simulink model "ECE724A"  (R2021b)
settings: Solver=ode3  StartTime=0.0  StopTime=sim_duration  FixedStep=0.01  RelTol=1e-3
model workspace: external: MAT-File C:\Users\jimmy\Desktop\61508010.mat (data not in the file)
undefined symbols (not defined in the file or in its folder): Base_power, columbeff, efficiency, efficiency_speed, efficiency_torque, f_d, f_tire_friction, f_tire_speed, g, gear_efficiency, Init_capacity, J_fd, J_motor, J_wheel, OCV, OCV_SOC, R_chg, R_dis, r_mass, Regen_fraction, Regen_speed, Road_grade, SOC_init, SOC_min, Stop_speed, Torque_curve_speed, Torque_curve_torque, Vehicle_weight, Wheel_radius
libraries: simulink x1
settings Model: Creator=jimmy  LastModifiedBy=jimmy

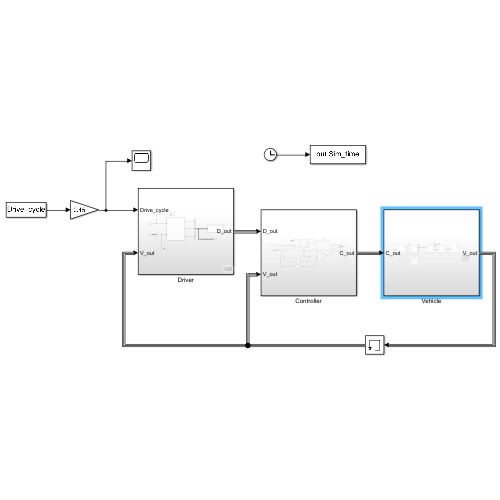
[thumbnail: Simulink's stored preview of the top-level diagram]
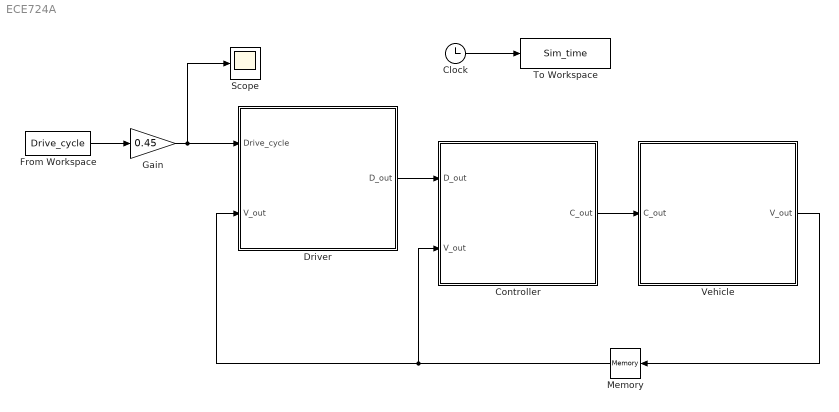
== system ECE724A ==
  Clock : Clock
  Controller : Subsystem
  Driver : Subsystem
  From Workspace : FromWorkspace  VariableName=Drive_cycle
  Gain : Gain  Gain=0.45
  Memory : Memory  InheritSampleTime=on  LinearizeMemory=on  LinearizeAsDelay=on
  Scope : Scope
  To Workspace : ToWorkspace  VariableName=Sim_time  SaveFormat=Timeseries  SampleTime=-1
  Vehicle : Subsystem
  wires:
  Vehicle/1(V_out) -> Memory/1
  Controller/1(C_out) -> Vehicle/1(C_out)
  Memory/1 -> Controller/2(V_out), Driver/2(V_out)
  Clock/1 -> To Workspace/1
  Driver/1(D_out) -> Controller/1(D_out)
  From Workspace/1 -> Gain/1
  Gain/1 -> Scope/1, Driver/1(Drive_cycle)

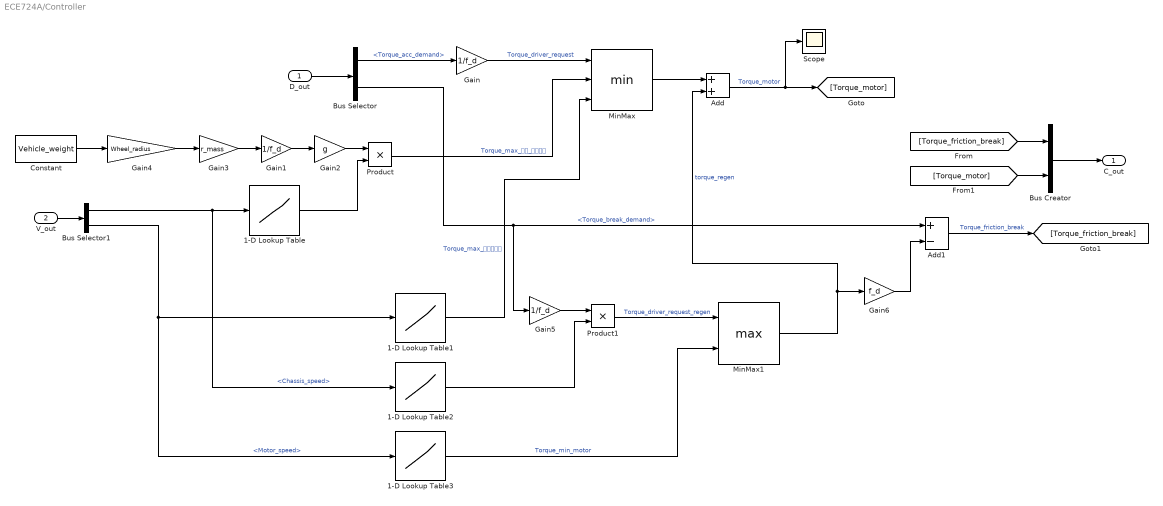
== system ECE724A/Controller ==
  D_out : Inport
  V_out : Inport  Port=2
  1-D Lookup Table : Lookup_n-D  NumberOfTableDimensions=1  BreakpointsForDimension1=f_tire_speed  Table=f_tire_friction  InternalRulePriority=Speed  RndMeth=Simplest  InputSameDT=on
  1-D Lookup Table1 : Lookup_n-D  NumberOfTableDimensions=1  BreakpointsForDimension1=Torque_curve_speed  Table=Torque_curve_torque  InternalRulePriority=Speed  RndMeth=Simplest  InputSameDT=on
  1-D Lookup Table2 : Lookup_n-D  NumberOfTableDimensions=1  BreakpointsForDimension1=Regen_speed  Table=Regen_fraction  InternalRulePriority=Speed  RndMeth=Simplest  InputSameDT=on
  1-D Lookup Table3 : Lookup_n-D  NumberOfTableDimensions=1  BreakpointsForDimension1=Torque_curve_speed  Table=-Torque_curve_torque  InternalRulePriority=Speed  RndMeth=Simplest  InputSameDT=on
  Add : Sum
  Add1 : Sum  Inputs=+-
  Bus Creator : BusCreator  Inputs=2
  Bus Selector : BusSelector  OutputSignals=Torque_acc_demand,Torque_break_demand
  Bus Selector1 : BusSelector  OutputSignals=Chassis.Chassis_speed,Motor.Motor_speed
  Constant : Constant  Value=Vehicle_weight
  Gain : Gain  Gain=1/f_d
  Gain1 : Gain  Gain=1/f_d
  Gain2 : Gain  Gain=g
  Gain3 : Gain  Gain=r_mass
  Gain4 : Gain  Gain=Wheel_radius
  Gain5 : Gain  Gain=1/f_d
  Gain6 : Gain  Gain=f_d
  MinMax : MinMax  Inputs=3
  MinMax1 : MinMax  Function=max  Inputs=2
  Product : Product
  Product1 : Product
  Scope : Scope
  C_out : Outport
  wires:
  D_out/1 -> Bus Selector/1
  Bus Selector/1 -> Gain/1  "<Torque_acc_demand>"
  Bus Selector/2 -> Gain5/1, Add1/1  "<Torque_break_demand>"
  Gain/1 -> MinMax/1  "Torque_driver_request"
  Constant/1 -> Gain4/1
  Gain4/1 -> Gain3/1
  Gain3/1 -> Gain1/1
  Gain1/1 -> Gain2/1
  1-D Lookup Table/1 -> Product/2
  Bus Selector1/1 -> 1-D Lookup Table2/1, 1-D Lookup Table/1  "<Chassis_speed>"
  Gain2/1 -> Product/1
  V_out/1 -> Bus Selector1/1
  Product/1 -> MinMax/2  "Torque_max_𝑛𝑜_𝑠𝑙𝑖𝑝"
  MinMax/1 -> Add/1
  Bus Selector1/2 -> 1-D Lookup Table3/1, 1-D Lookup Table1/1  "<Motor_speed>"
  1-D Lookup Table1/1 -> MinMax/3  "Torque_max_𝑚𝑜𝑡𝑜𝑟"
  Gain5/1 -> Product1/1
  1-D Lookup Table2/1 -> Product1/2
  Product1/1 -> MinMax1/1  "Torque_driver_request_regen"
  1-D Lookup Table3/1 -> MinMax1/2  "Torque_min_motor"
  MinMax1/1 -> Gain6/1, Add/2  "torque_regen"
  Add/1 -> Scope/1, [Torque_motor]  "Torque_motor"
  Gain6/1 -> Add1/2
  Add1/1 -> [Torque_friction_break]  "Torque_friction_break"
  [Torque_motor] -> Bus Creator/2
  [Torque_friction_break] -> Bus Creator/1
  Bus Creator/1 -> C_out/1

== system ECE724A/Driver ==
  Drive_cycle : Inport
  V_out : Inport  Port=2
  Bus Creator : BusCreator  Inputs=3
  Bus Selector : BusSelector  OutputSignals=Chassis.Chassis_speed
  Plant : Subsystem
  Scope : Scope
  Scope1 : Scope
  To workspace : Subsystem
  D_out : Outport
  wires:
  Drive_cycle/1 -> Scope/1, Plant/1(Drive_cycle)
  V_out/1 -> Bus Selector/1
  Bus Selector/1 -> Scope1/1, Plant/2(Chasis_speed)  "<Chassis_speed>"
  Plant/1(Linear_speed_demand) -> Bus Creator/1
  Plant/2(Torque_acc_demand) -> Bus Creator/2
  Plant/3(Torque_break_demand) -> Bus Creator/3
  Bus Creator/1 -> D_out/1, To workspace/1(In1)

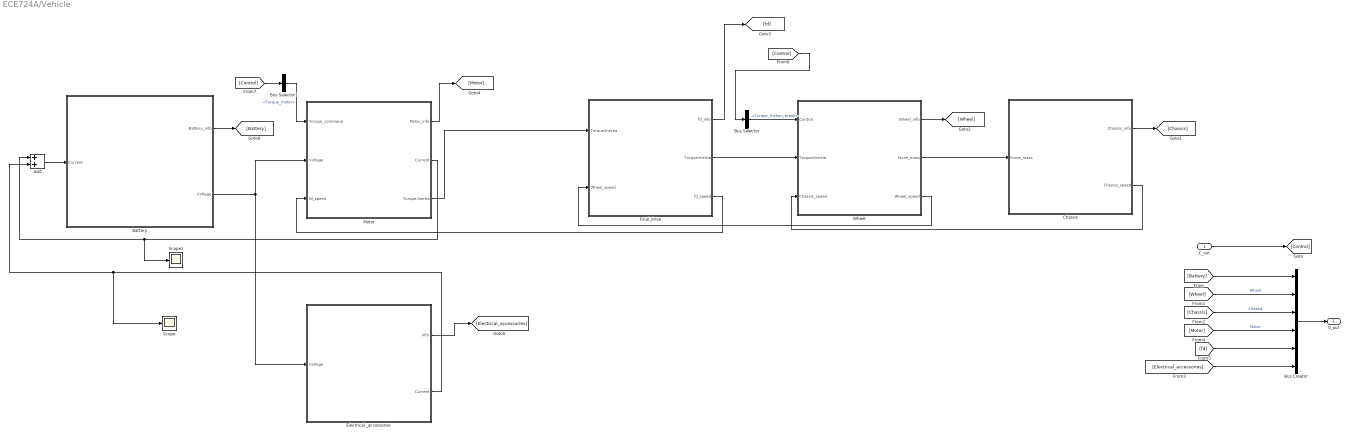
== system ECE724A/Vehicle ==
  C_out : Inport
  Add : Sum
  Battery : Subsystem
  Bus Creator : BusCreator  Inputs=6
  Bus Selector : BusSelector  OutputSignals=Torque_friction_break
  Bus Selector1 : BusSelector  OutputSignals=Torque_motor
  Chassis : Subsystem
  Electrical _accessories : Subsystem
  Final_drive : Subsystem
  Motor : Subsystem
  Scope : Scope
  Scope1 : Scope
  Wheel : Subsystem
  V_out : Outport
  wires:
  Bus Creator/1 -> V_out/1
  [Battery] -> Bus Creator/1
  [Wheel] -> Bus Creator/2  "Wheel"
  [Chassis] -> Bus Creator/3  "Chassis"
  [Motor] -> Bus Creator/4  "Motor"
  [fd] -> Bus Creator/5
  [Electrical_accessories] -> Bus Creator/6
  C_out/1 -> [Control]
  Chassis/1(Chassis_info) -> [Chassis]
  Wheel/2(Force_mass) -> Chassis/1(Force_mass)
  Wheel/1(Wheel_info) -> [Wheel]
  Chassis/2(Chassis_speed) -> Wheel/3(Chassis_speed)
  Final_drive/2(Torque/Inertia) -> Wheel/2(Torque/Inertia)
  Wheel/3(Wheel_speed) -> Final_drive/2(Wheel_speed)
  Final_drive/3(fd_speed) -> Motor/3(fd_speed)
  Motor/3("Torque/Inertia ") -> Final_drive/1("Torque/Inertia ")
  Final_drive/1(fd_info) -> [fd]
  Battery/2(Voltage) -> Motor/2(Voltage), Electrical _accessories/1(Voltage)
  Motor/2(Current) -> Scope1/1, Add/1
  Motor/1(Motor_info) -> [Motor]
  Bus Selector/1 -> Wheel/1(Control)  "<Torque_friction_break>"
  [Control] -> Bus Selector/1
  [Control] -> Bus Selector1/1
  Bus Selector1/1 -> Motor/1(Torque_command)  "<Torque_motor>"
  Add/1 -> Battery/1(Current)
  Electrical _accessories/2(Current) -> Scope/1, Add/2
  Electrical _accessories/1(Info) -> [Electrical_accessories]
  Battery/1(Battery_info) -> [Battery]

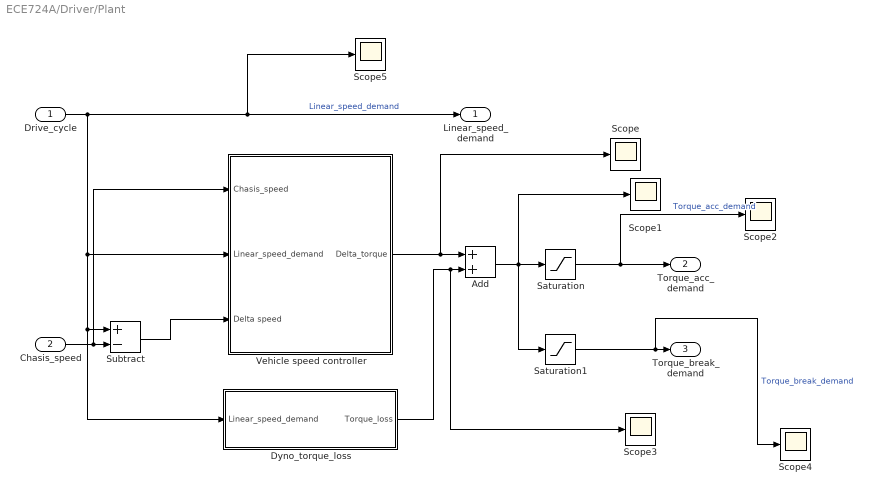
== system ECE724A/Driver/Plant ==
  Drive_cycle : Inport
  Chasis_speed : Inport  Port=2
  Add : Sum
  Dyno_torque_loss : Subsystem
  Saturation : Saturate  UpperLimit=inf  LowerLimit=0
  Saturation1 : Saturate  UpperLimit=0  LowerLimit=-inf
  Scope{,1..5} (6 alike) : Scope
  Subtract : Sum  Inputs=+-
  Vehicle speed controller : Subsystem
  Linear_speed_demand : Outport
  Torque_acc_demand : Outport  Port=2
  Torque_break_demand : Outport  Port=3
  wires:
  Drive_cycle/1 -> Vehicle speed controller/2(Linear_speed_demand), Dyno_torque_loss/1(Linear_speed_demand), Subtract/1, Scope5/1, Linear_speed_demand/1  "Linear_speed_demand"
  Chasis_speed/1 -> Vehicle speed controller/1(Chasis_speed), Subtract/2
  Subtract/1 -> Vehicle speed controller/3(Delta speed)
  Vehicle speed controller/1(Delta_torque) -> Scope/1, Add/1
  Dyno_torque_loss/1(Torque_loss) -> Scope3/1, Add/2
  Add/1 -> Saturation1/1, Scope1/1, Saturation/1
  Saturation/1 -> Scope2/1, Torque_acc_demand/1  "Torque_acc_demand"
  Saturation1/1 -> Scope4/1, Torque_break_demand/1  "Torque_break_demand"

== system ECE724A/Driver/To workspace ==
  In1 : Inport
  Bus Selector : BusSelector  OutputSignals=Linear_speed_demand,Torque_acc_demand,Torque_break_demand
  To Workspace : ToWorkspace  VariableName=Linear_speed_demand  SampleTime=0.1
      settings: Decimation=10  Save2DSignal=2-D array (concatenate along first dimension)
  To Workspace2 : ToWorkspace  VariableName=Torque_break_demand  SampleTime=-1
      settings: Decimation=10
  To Workspace3 : ToWorkspace  VariableName=Torque_acc_demand  SampleTime=-1
      settings: Decimation=10
  wires:
  In1/1 -> Bus Selector/1
  Bus Selector/1 -> To Workspace/1  "<Linear_speed_demand>"
  Bus Selector/2 -> To Workspace3/1  "<Torque_acc_demand>"
  Bus Selector/3 -> To Workspace2/1  "<Torque_break_demand>"

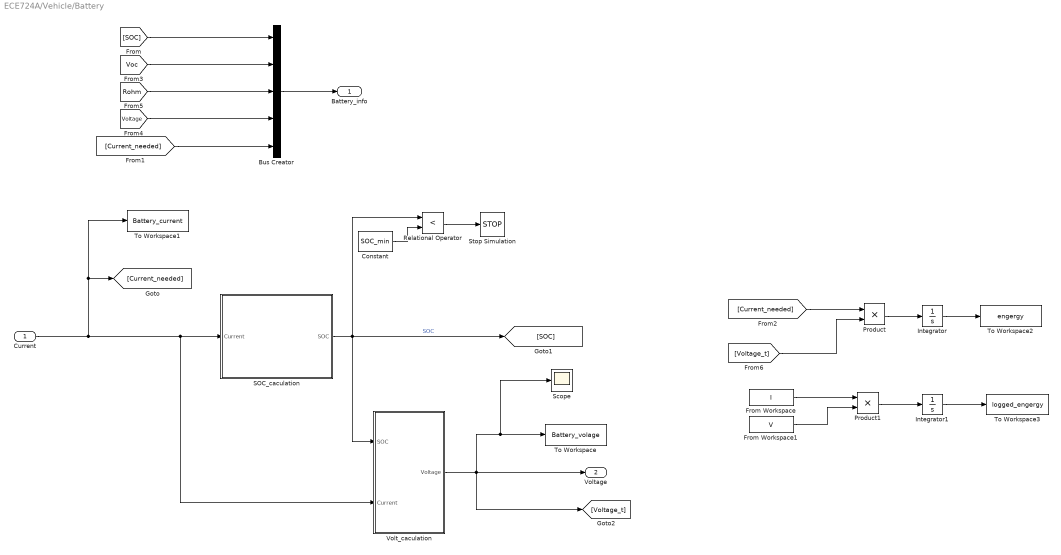
== system ECE724A/Vehicle/Battery ==
  Current : Inport
  Bus Creator : BusCreator  Inputs=5
  Constant : Constant  Value=SOC_min
  From Workspace : FromWorkspace  VariableName=I
  From Workspace1 : FromWorkspace  VariableName=V
  Integrator : Integrator
  Integrator1 : Integrator
  Product : Product
  Product1 : Product
  Relational Operator : RelationalOperator  Operator=<  OutDataTypeStr=boolean  RndMeth=Simplest
  SOC_caculation : Subsystem
  Scope : Scope
  Stop Simulation : Stop
  To Workspace : ToWorkspace  VariableName=Battery_volage  SampleTime=0.1
  To Workspace1 : ToWorkspace  VariableName=Battery_current  SampleTime=0.1
  To Workspace2 : ToWorkspace  VariableName=engergy  SampleTime=-1
  To Workspace3 : ToWorkspace  VariableName=logged_engergy  SampleTime=-1
  Volt_caculation : Subsystem
  Battery_info : Outport
  Voltage : Outport  Port=2
  wires:
  Current/1 -> To Workspace1/1, [Current_needed], Volt_caculation/2(Current), SOC_caculation/1(Current)
  SOC_caculation/1(SOC) -> Volt_caculation/1(SOC), Relational Operator/1, [SOC]  "SOC"
  Constant/1 -> Relational Operator/2
  Relational Operator/1 -> Stop Simulation/1
  Volt_caculation/1(Voltage) -> [Voltage_t], Scope/1, To Workspace/1, Voltage/1
  Bus Creator/1 -> Battery_info/1
  [Current_needed] -> Bus Creator/5
  [SOC] -> Bus Creator/1
  [Voc] -> Bus Creator/2
  [Rohm] -> Bus Creator/3
  [Voltage] -> Bus Creator/4
  [Voltage_t] -> Product/2
  [Current_needed] -> Product/1
  Product/1 -> Integrator/1
  Integrator/1 -> To Workspace2/1
  From Workspace/1 -> Product1/1
  From Workspace1/1 -> Product1/2
  Product1/1 -> Integrator1/1
  Integrator1/1 -> To Workspace3/1

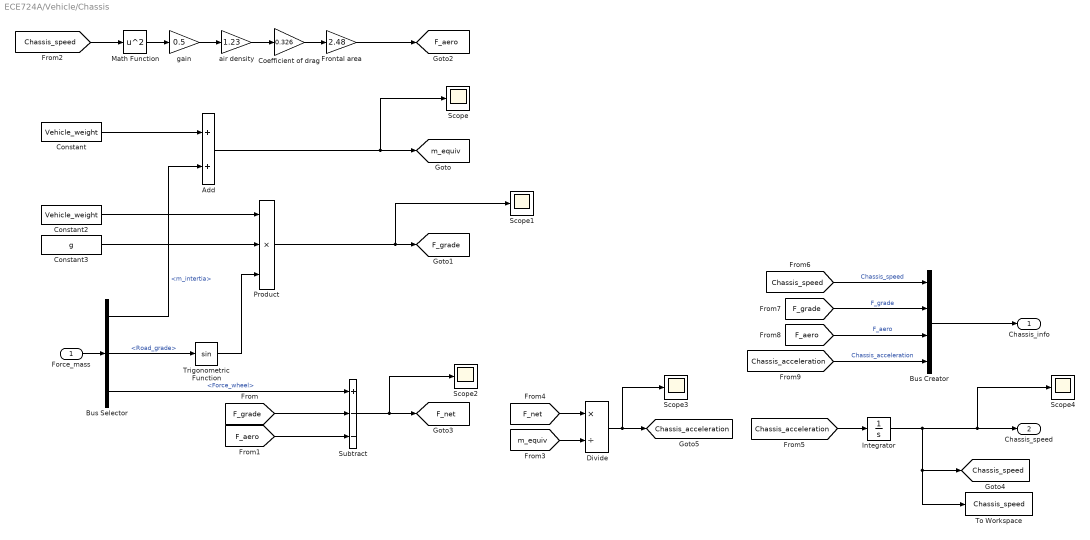
== system ECE724A/Vehicle/Chassis ==
  Force_mass : Inport
  Add : Sum
  Bus Creator : BusCreator  Inputs=4
  Bus Selector : BusSelector  OutputSignals=m_intertia,Road_grade,Force_wheel
  Coefficient of drag : Gain  Gain=0.326
  Constant : Constant  Value=Vehicle_weight
  Constant2 : Constant  Value=Vehicle_weight
  Constant3 : Constant  Value=g
  Divide : Product  Inputs=*/
  Frontal area : Gain  Gain=2.48
  Integrator : Integrator
  Math Function : Math  Operator=square  SaturateOnIntegerOverflow=on
  Product : Product  Inputs=3
  Scope{,1..4} (5 alike) : Scope
  Subtract : Sum  Inputs=+--
  To Workspace : ToWorkspace  VariableName=Chassis_speed  SampleTime=0.1
  Trigonometric Function : Trigonometry
  air density : Gain  Gain=1.23
  gain : Gain  Gain=0.5
  Chassis_info : Outport
  Chassis_speed : Outport  Port=2
  tag scope: Chassis_acceleration=global, Chassis_speed=global, F_aero=global, F_grade=global, F_net=global, m_equiv=global
  wires:
  Force_mass/1 -> Bus Selector/1
  Integrator/1 -> To Workspace/1, [Chassis_speed], Scope4/1, Chassis_speed/1
  [Chassis_acceleration] -> Integrator/1
  [F_net] -> Divide/1
  [m_equiv] -> Divide/2
  Divide/1 -> Scope3/1, [Chassis_acceleration]
  Constant/1 -> Add/1
  Add/1 -> Scope/1, [m_equiv]
  Bus Selector/1 -> Add/2  "<m_intertia>"
  Bus Selector/2 -> Trigonometric Function/1  "<Road_grade>"
  Trigonometric Function/1 -> Product/3
  Product/1 -> Scope1/1, [F_grade]
  Bus Selector/3 -> Subtract/1  "<Force_wheel>"
  [F_grade] -> Subtract/2
  gain/1 -> air density/1
  air density/1 -> Coefficient of drag/1
  Coefficient of drag/1 -> Frontal area/1
  Frontal area/1 -> [F_aero]
  [Chassis_speed] -> Math Function/1
  Math Function/1 -> gain/1
  [F_aero] -> Subtract/3
  Subtract/1 -> Scope2/1, [F_net]
  [Chassis_speed] -> Bus Creator/1  "Chassis_speed"
  [F_grade] -> Bus Creator/2  "F_grade"
  [F_aero] -> Bus Creator/3  "F_aero"
  [Chassis_acceleration] -> Bus Creator/4  "Chassis_acceleration"
  Bus Creator/1 -> Chassis_info/1
  Constant3/1 -> Product/2
  Constant2/1 -> Product/1

== system ECE724A/Vehicle/Electrical _accessories ==
  Voltage : Inport
  Constant : Constant  Value=Base_power
  Divider : Subsystem
  Info : Outport
  Current : Outport  Port=2
  wires:
  Divider/1(Out1) -> Current/1
  Constant/1 -> Divider/1(Current)
  Voltage/1 -> Divider/2(Voltage)

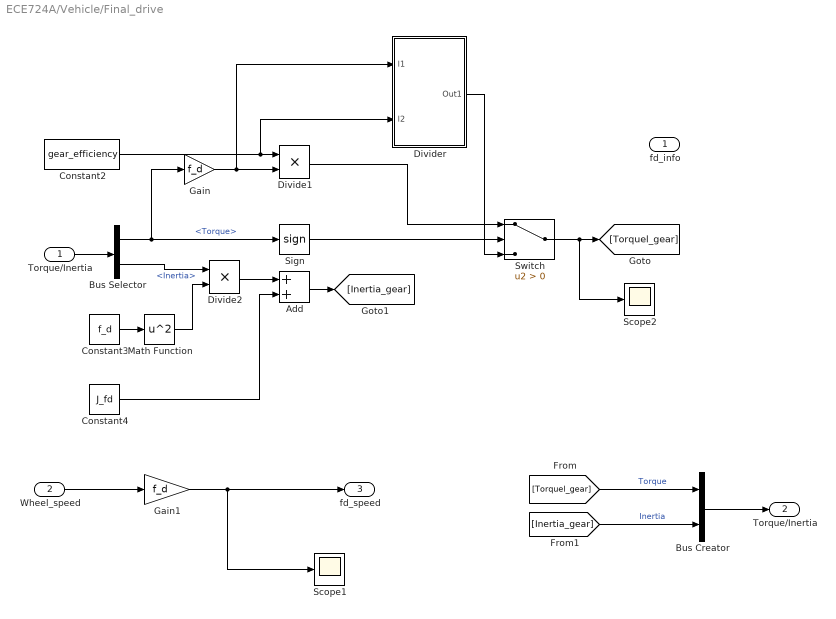
== system ECE724A/Vehicle/Final_drive ==
  "Torque/Inertia " : Inport
  Wheel_speed : Inport  Port=2
  Add : Sum
  Bus Creator : BusCreator  Inputs=2
  Bus Selector : BusSelector  OutputSignals=Torque,Inertia
  Constant2 : Constant  Value=gear_efficiency
  Constant3 : Constant  Value=f_d
  Constant4 : Constant  Value=J_fd
  Divide1 : Product  Inputs=**
  Divide2 : Product  Inputs=**
  Divider : Subsystem
  Gain : Gain  Gain=f_d
  Gain1 : Gain  Gain=f_d
  Math Function : Math  Operator=square  SaturateOnIntegerOverflow=on
  Scope1 : Scope
  Scope2 : Scope
  Sign : Signum
  Switch : Switch  Criteria=u2 > Threshold
  fd_info : Outport
  Torque/Inertia : Outport  Port=2
  fd_speed : Outport  Port=3
  wires:
  [Torquel_gear] -> Bus Creator/1  "Torque"
  [Inertia_gear] -> Bus Creator/2  "Inertia"
  Bus Creator/1 -> Torque/Inertia/1
  Wheel_speed/1 -> Gain1/1
  "Torque/Inertia "/1 -> Bus Selector/1
  Bus Selector/1 -> Sign/1, Gain/1  "<Torque>"
  Constant2/1 -> Divider/2(l2), Divide1/1
  Constant3/1 -> Math Function/1
  Bus Selector/2 -> Divide2/1  "<Inertia>"
  Math Function/1 -> Divide2/2
  Divide2/1 -> Add/1
  Constant4/1 -> Add/2
  Add/1 -> [Inertia_gear]
  Sign/1 -> Switch/2
  Switch/1 -> Scope2/1, [Torquel_gear]
  Divide1/1 -> Switch/1
  Divider/1(Out1) -> Switch/3
  Gain/1 -> Divide1/2, Divider/1(l1)
  Gain1/1 -> Scope1/1, fd_speed/1

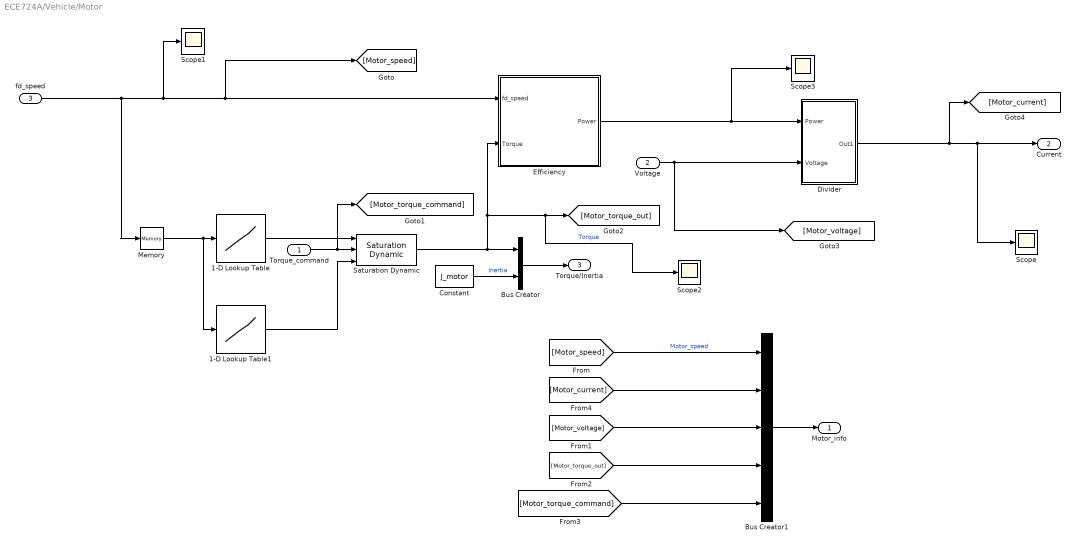
== system ECE724A/Vehicle/Motor ==
  Torque_command : Inport
  Voltage : Inport  Port=2
  fd_speed : Inport  Port=3
  1-D Lookup Table : Lookup_n-D  NumberOfTableDimensions=1  BreakpointsForDimension1=Torque_curve_speed  Table=Torque_curve_torque  InternalRulePriority=Speed  RndMeth=Simplest  InputSameDT=on
  1-D Lookup Table1 : Lookup_n-D  NumberOfTableDimensions=1  BreakpointsForDimension1=Torque_curve_speed  Table=-Torque_curve_torque  InternalRulePriority=Speed  RndMeth=Simplest  InputSameDT=on
  Bus Creator : BusCreator  Inputs=2
  Bus Creator1 : BusCreator  Inputs=5
  Constant : Constant  Value=J_motor
  Divider : Subsystem
  Efficiency : Subsystem
  Memory : Memory  InheritSampleTime=on  LinearizeMemory=on  LinearizeAsDelay=on
  Saturation Dynamic : simulink/Discontinuities/Saturation Dynamic  OutMin=[]  OutMax=[]  OutDataTypeStr=Inherit: Same as second input  OutDataType=fixdt(1, 16)  OutScaling=2^-10  DoSatur=off
  Scope{,1..3} (4 alike) : Scope
  Motor_info : Outport
  Current : Outport  Port=2
  "Torque/Inertia " : Outport  Port=3
  wires:
  Bus Creator/1 -> "Torque/Inertia "/1
  Constant/1 -> Bus Creator/2  "Inertia"
  Saturation Dynamic/1 -> Efficiency/2(Torque), Scope2/1, [Motor_torque_out], Bus Creator/1  "Torque"
  Memory/1 -> 1-D Lookup Table1/1, 1-D Lookup Table/1
  1-D Lookup Table/1 -> Saturation Dynamic/1
  1-D Lookup Table1/1 -> Saturation Dynamic/3
  Torque_command/1 -> [Motor_torque_command], Saturation Dynamic/2
  Voltage/1 -> [Motor_voltage], Divider/2(Voltage)
  Efficiency/1(Power) -> Scope3/1, Divider/1(Power)
  Bus Creator1/1 -> Motor_info/1
  [Motor_speed] -> Bus Creator1/1  "Motor_speed"
  [Motor_current] -> Bus Creator1/2
  [Motor_voltage] -> Bus Creator1/3
  [Motor_torque_out] -> Bus Creator1/4
  [Motor_torque_command] -> Bus Creator1/5
  fd_speed/1 -> Memory/1, Scope1/1, Efficiency/1(fd_speed), [Motor_speed]
  Divider/1(Out1) -> [Motor_current], Scope/1, Current/1

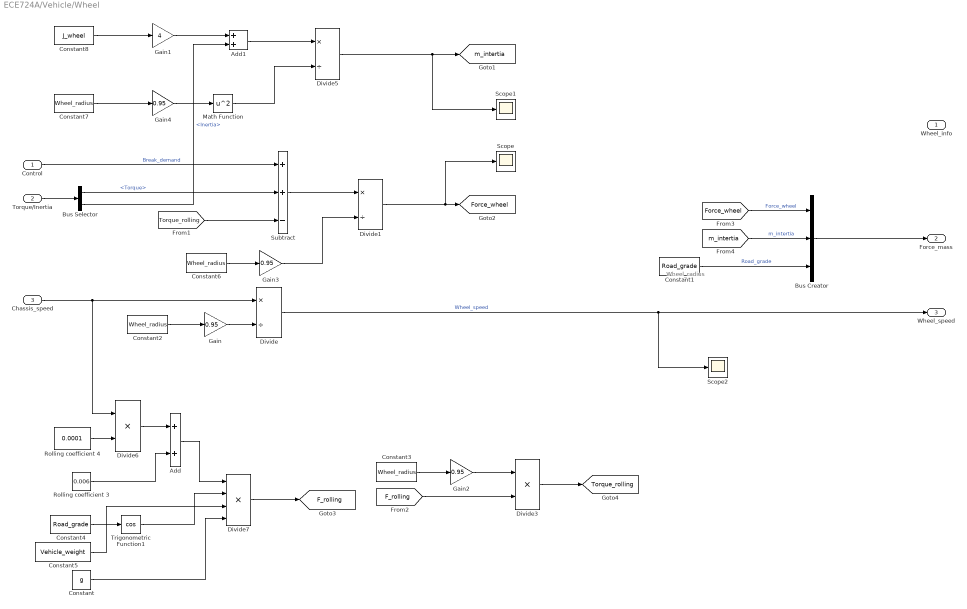
== system ECE724A/Vehicle/Wheel ==
  note: Wheel_radius
  Control : Inport
  Torque/Inertia : Inport  Port=2
  Chassis_speed : Inport  Port=3
  Add : Sum
  Add1 : Sum
  Bus Creator : BusCreator  Inputs=3
  Bus Selector : BusSelector  OutputSignals=Torque,Inertia
  Constant : Constant  Value=g
  Constant1 : Constant  Value=Road_grade
  Constant{2..3,6..7} (4 alike) : Constant  Value=Wheel_radius
  Constant4 : Constant  Value=Road_grade
  Constant5 : Constant  Value=Vehicle_weight
  Constant8 : Constant  Value=J_wheel
  Divide : Product  Inputs=*/
  Divide1 : Product  Inputs=*/
  Divide3 : Product  Inputs=**
  Divide5 : Product  Inputs=*/
  Divide6 : Product  Inputs=**
  Divide7 : Product  Inputs=****
  Gain{,2..4} (4 alike) : Gain  Gain=0.95
  Gain1 : Gain  Gain=4
  Math Function : Math  Operator=square  SaturateOnIntegerOverflow=on
  Rolling coefficient 3 : Constant  Value=0.006
  Rolling coefficient 4 : Constant  Value=0.0001
  Scope : Scope
  Scope1 : Scope
  Scope2 : Scope
  Subtract : Sum  Inputs=++-
  Trigonometric Function1 : Trigonometry  Operator=cos
  Wheel_info : Outport
  Force_mass : Outport  Port=2
  Wheel_speed : Outport  Port=3
  tag scope: F_rolling=global, Force_wheel=global, Torque_rolling=global, m_intertia=global
  wires:
  Bus Creator/1 -> Force_mass/1
  [Force_wheel] -> Bus Creator/1  "Force_wheel"
  [m_intertia] -> Bus Creator/2  "m_intertia"
  Constant1/1 -> Bus Creator/3  "Road_grade"
  Chassis_speed/1 -> Divide6/1, Divide/1
  Divide/1 -> Scope2/1, Wheel_speed/1  "Wheel_speed"
  Control/1 -> Subtract/1  "Break_demand"
  [Torque_rolling] -> Subtract/3
  Subtract/1 -> Divide1/1
  Divide1/1 -> Scope/1, [Force_wheel]
  Constant8/1 -> Gain1/1
  Gain1/1 -> Add1/1
  Add1/1 -> Divide5/1
  Math Function/1 -> Divide5/2
  Divide5/1 -> Scope1/1, [m_intertia]
  Rolling coefficient 4/1 -> Divide6/2
  Divide6/1 -> Add/1
  Rolling coefficient 3/1 -> Add/2
  Add/1 -> Divide7/1
  Constant4/1 -> Trigonometric Function1/1
  Trigonometric Function1/1 -> Divide7/2
  Constant5/1 -> Divide7/3
  Constant/1 -> Divide7/4
  Divide7/1 -> [F_rolling]
  [F_rolling] -> Divide3/2
  Constant3/1 -> Gain2/1
  Divide3/1 -> [Torque_rolling]
  Gain2/1 -> Divide3/1
  Constant2/1 -> Gain/1
  Gain/1 -> Divide/2
  Constant6/1 -> Gain3/1
  Gain3/1 -> Divide1/2
  Constant7/1 -> Gain4/1
  Gain4/1 -> Math Function/1
  Torque/Inertia/1 -> Bus Selector/1
  Bus Selector/1 -> Subtract/2  "<Torque>"
  Bus Selector/2 -> Add1/2  "<Inertia>"

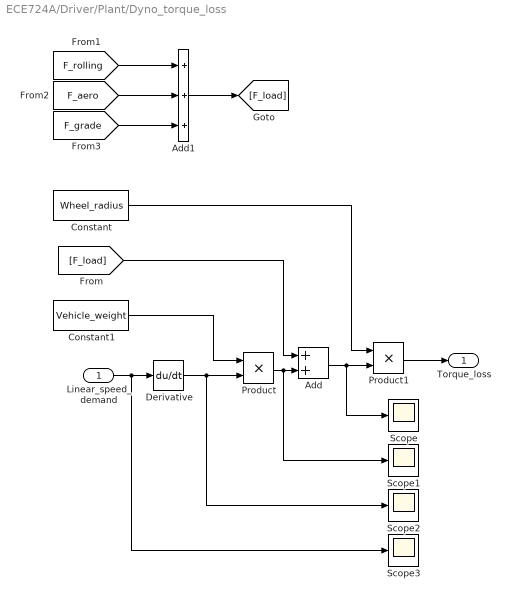
== system ECE724A/Driver/Plant/Dyno_torque_loss ==
  Linear_speed_demand : Inport
  Add : Sum
  Add1 : Sum  Inputs=+++
  Constant : Constant  Value=Wheel_radius
  Constant1 : Constant  Value=Vehicle_weight
  Derivative : Derivative
  Product : Product
  Product1 : Product
  Scope{,1..3} (4 alike) : Scope
  Torque_loss : Outport
  wires:
  Linear_speed_demand/1 -> Scope3/1, Derivative/1
  Derivative/1 -> Scope2/1, Product/2
  Constant1/1 -> Product/1
  Product/1 -> Scope1/1, Add/2
  [F_load] -> Add/1
  Add/1 -> Scope/1, Product1/2
  Constant/1 -> Product1/1
  Product1/1 -> Torque_loss/1
  [F_rolling] -> Add1/1
  [F_aero] -> Add1/2
  [F_grade] -> Add1/3
  Add1/1 -> [F_load]

== system ECE724A/Driver/Plant/Vehicle speed controller ==
  Chasis_speed : Inport
  Linear_speed_demand : Inport  Port=2
  Delta speed : Inport  Port=3
  Add : Sum
  Constant : Constant  Value=Stop_speed
  I : Gain  Gain=0.5
  Integrator : Integrator  ExternalReset=either
  P : Gain  Gain=1000
  Relational Operator : RelationalOperator  Operator=<  OutDataTypeStr=boolean  RndMeth=Simplest
  Delta_torque : Outport
  wires:
  Delta speed/1 -> P/1, Integrator/1
  Chasis_speed/1 -> Relational Operator/1
  Constant/1 -> Relational Operator/2
  Relational Operator/1 -> Integrator/2
  Integrator/1 -> I/1
  P/1 -> Add/1
  I/1 -> Add/2
  Add/1 -> Delta_torque/1  "Delta_torque"

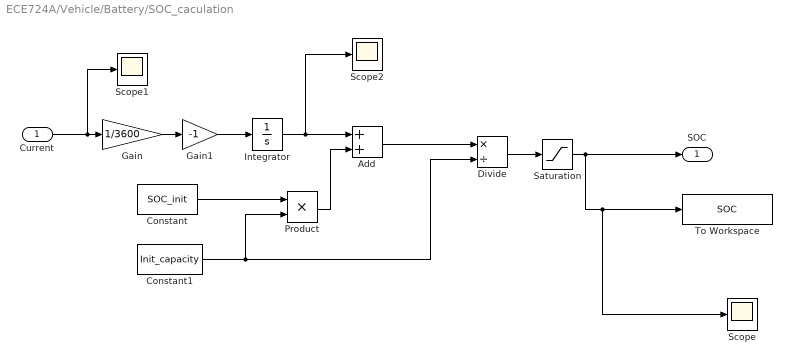
== system ECE724A/Vehicle/Battery/SOC_caculation ==
  Current : Inport
  Add : Sum
  Constant : Constant  Value=SOC_init
  Constant1 : Constant  Value=Init_capacity
  Divide : Product  Inputs=*/
  Gain : Gain  Gain=1/3600
  Gain1 : Gain  Gain=-1
  Integrator : Integrator
  Product : Product
  Saturation : Saturate  UpperLimit=1  LowerLimit=0
  Scope : Scope
  Scope1 : Scope
  Scope2 : Scope
  To Workspace : ToWorkspace  VariableName=SOC  SampleTime=0.1
  SOC : Outport
  wires:
  Gain/1 -> Gain1/1
  Current/1 -> Scope1/1, Gain/1
  Gain1/1 -> Integrator/1
  Constant/1 -> Product/1
  Constant1/1 -> Divide/2, Product/2
  Divide/1 -> Saturation/1
  Add/1 -> Divide/1
  Integrator/1 -> Scope2/1, Add/1
  Product/1 -> Add/2
  Saturation/1 -> Scope/1, To Workspace/1, SOC/1

== system ECE724A/Vehicle/Battery/Volt_caculation ==
  SOC : Inport
  Current : Inport  Port=2
  1-D Lookup Table : Lookup_n-D  NumberOfTableDimensions=1  BreakpointsForDimension1=OCV_SOC  Table=OCV  InternalRulePriority=Speed  RndMeth=Simplest  InputSameDT=on
  1-D Lookup Table1 : Lookup_n-D  NumberOfTableDimensions=1  BreakpointsForDimension1=OCV_SOC  Table=R_chg  InternalRulePriority=Speed  RndMeth=Simplest  InputSameDT=on
  1-D Lookup Table2 : Lookup_n-D  NumberOfTableDimensions=1  BreakpointsForDimension1=OCV_SOC  Table=R_dis  InternalRulePriority=Speed  RndMeth=Simplest  InputSameDT=on
  Gain : Gain  Gain=columbeff
  Product1 : Product
  Subtract : Sum  Inputs=+-
  Switch : Switch  Criteria=u2 > Threshold
  Switch1 : Switch  Criteria=u2 > Threshold
  Voltage : Outport
  tag scope: Rohm=global, Voc=global, Voltage=global
  wires:
  SOC/1 -> 1-D Lookup Table1/1, 1-D Lookup Table2/1, 1-D Lookup Table/1
  1-D Lookup Table/1 -> Subtract/1, [Voc]
  1-D Lookup Table2/1 -> Switch/3
  1-D Lookup Table1/1 -> Switch/1
  Switch/1 -> Product1/2, [Rohm]
  Switch1/1 -> Product1/1, Switch/2
  Current/1 -> Switch1/2, Switch1/1, Gain/1
  Gain/1 -> Switch1/3
  Product1/1 -> Subtract/2
  Subtract/1 -> [Voltage]
  [Voltage] -> Voltage/1

== system ECE724A/Vehicle/Electrical _accessories/Divider ==
  Current : Inport
  Voltage : Inport  Port=2
  Bus Creator : BusCreator  Inputs=2
  Interpreted MATLAB Function : MATLABFcn  MATLABFcn=myFunction
  Out1 : Outport
  wires:
  Current/1 -> Bus Creator/1
  Voltage/1 -> Bus Creator/2
  Bus Creator/1 -> Interpreted MATLAB Function/1
  Interpreted MATLAB Function/1 -> Out1/1

== system ECE724A/Vehicle/Final_drive/Divider ==
  l1 : Inport
  l2 : Inport  Port=2
  Bus Creator : BusCreator  Inputs=2
  Interpreted MATLAB Function : MATLABFcn  MATLABFcn=myFunction
  Out1 : Outport
  wires:
  l1/1 -> Bus Creator/1
  l2/1 -> Bus Creator/2
  Bus Creator/1 -> Interpreted MATLAB Function/1
  Interpreted MATLAB Function/1 -> Out1/1

== system ECE724A/Vehicle/Motor/Divider ==
  Power : Inport
  Voltage : Inport  Port=2
  Bus Creator : BusCreator  Inputs=2
  Interpreted MATLAB Function : MATLABFcn  MATLABFcn=myFunction
  Out1 : Outport
  wires:
  Power/1 -> Bus Creator/1
  Voltage/1 -> Bus Creator/2
  Bus Creator/1 -> Interpreted MATLAB Function/1
  Interpreted MATLAB Function/1 -> Out1/1

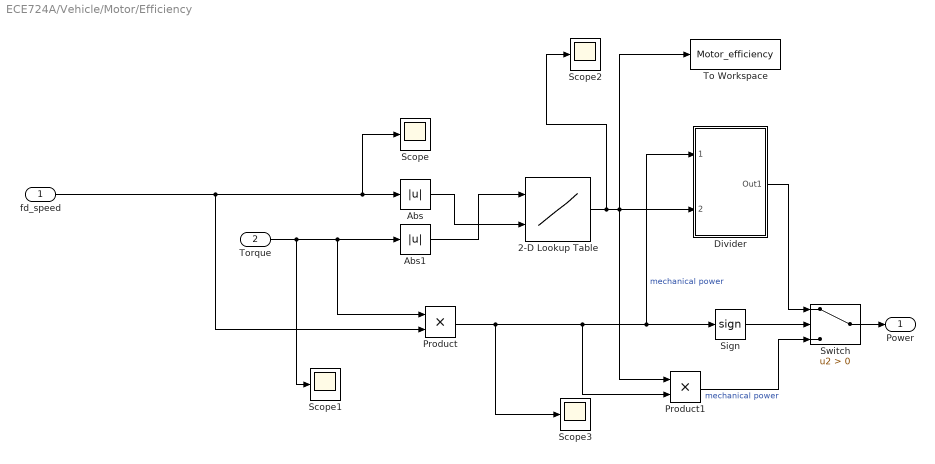
== system ECE724A/Vehicle/Motor/Efficiency ==
  fd_speed : Inport
  Torque : Inport  Port=2
  2-D Lookup Table : Lookup_n-D  BreakpointsForDimension1=efficiency_torque  BreakpointsForDimension2=efficiency_speed  Table=efficiency  InternalRulePriority=Speed  RndMeth=Simplest  InputSameDT=on
      settings: InputPortMap=u0,u1
  Abs : Abs
  Abs1 : Abs
  Divider : Subsystem
  Product : Product
  Product1 : Product
  Scope{,1..3} (4 alike) : Scope
  Sign : Signum
  Switch : Switch  Criteria=u2 > Threshold
  To Workspace : ToWorkspace  VariableName=Motor_efficiency  SaveFormat=Timeseries  SampleTime=-1
  Power : Outport
  wires:
  Torque/1 -> Scope1/1, Product/1, Abs1/1
  Product/1 -> Scope3/1, Product1/2, Divider/1(1), Sign/1  "mechanical power"
  Sign/1 -> Switch/2
  Switch/1 -> Power/1
  2-D Lookup Table/1 -> Scope2/1, Product1/1, To Workspace/1, Divider/2(2)
  Product1/1 -> Switch/3  "mechanical power"
  Divider/1(Out1) -> Switch/1
  Abs1/1 -> 2-D Lookup Table/1
  Abs/1 -> 2-D Lookup Table/2
  fd_speed/1 -> Scope/1, Abs/1, Product/2

== system ECE724A/Vehicle/Motor/Efficiency/Divider ==
  1 : Inport
  2 : Inport  Port=2
  Bus Creator : BusCreator  Inputs=2
  Interpreted MATLAB Function : MATLABFcn  MATLABFcn=myFunction
  Out1 : Outport
  wires:
  1/1 -> Bus Creator/1
  2/1 -> Bus Creator/2
  Bus Creator/1 -> Interpreted MATLAB Function/1
  Interpreted MATLAB Function/1 -> Out1/1
